simulink model "blimp_state_space"  (R2024b)
settings: Solver=ode113  StartTime=0.0  StopTime=50  RelTol=1e-3
values from neighbouring files (symbols this model uses):
  param = init_params()    [blimp_sim.m]
libraries: slpidlib x1
settings Model: Creator=naikveda
settings SolverCC: SolverResetMethod=Robust

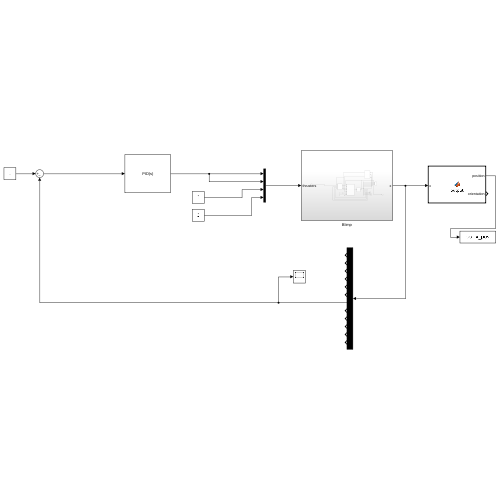
[thumbnail: Simulink's stored preview of the top-level diagram]
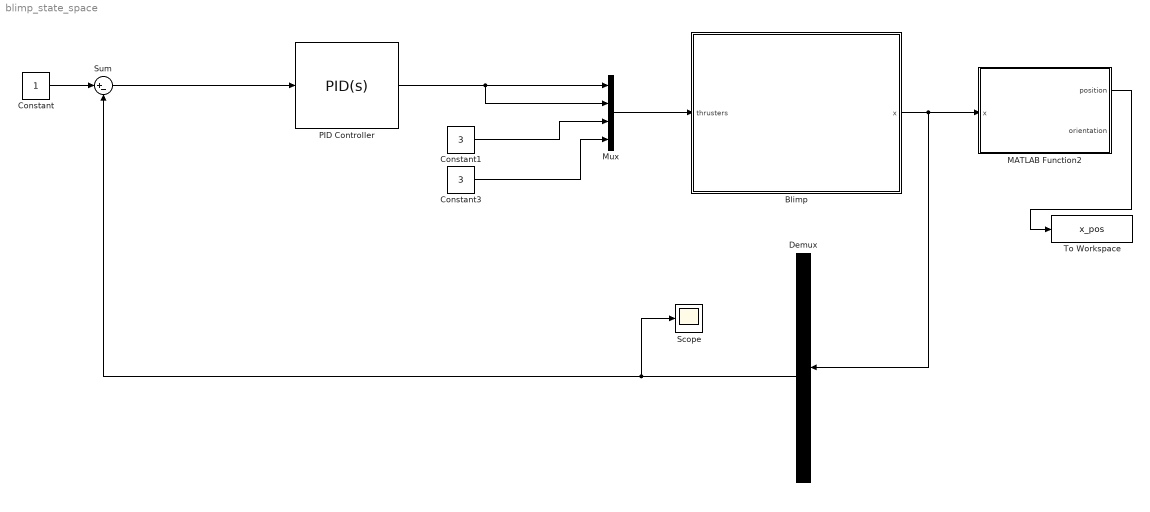
== system blimp_state_space ==
  Blimp : Subsystem
  Constant : Constant
  Constant1 : Constant  Value=3
  Constant3 : Constant  Value=3
  Demux : Demux  Outputs=12
  MATLAB Function2 : MATLAB Function  TreatAsAtomicUnit=on
  Mux : Mux
  PID Controller : slpidlib/PID Controller  Controller=PID  Form=Parallel  TimeDomain=Continuous-time  UseExternalTs=off  SampleTime=-1  IntegratorMethod=Forward Euler  FilterMethod=Forward Euler  ControllerParametersSource=internal  P=1  I=1  UseKiTs=off  D=0  UseExternalDerivativeSource=off  N=100  UseFilter=on  TunerSelectOption=Transfer Function Based (PID Tuner App)  InitialConditionSource=internal  InitialConditionForIntegrator=0  InitialConditionForFilter=0  DifferentiatorICPrevScaledInput=0  ExternalReset=none  TrackingMode=off  Kt=1  LimitOutput=off  SatLimitsSource=internal  UpperSaturationLimit=inf  LowerSaturationLimit=-inf  LinearizeAsGain=on  AntiWindupMode=none  Kb=1  LimitIntegrator=off  UpperIntegratorSaturationLimit=inf  LowerIntegratorSaturationLimit=-inf  POutMin=[]  POutMax=[]  IOutMin=[]  IOutMax=[]  DOutMin=[]  DOutMax=[]  NOutMin=[]  NOutMax=[]  SumOutMin=[]  SumOutMax=[]  SaturationOutMin=[]  SaturationOutMax=[]  PParamMin=[]  PParamMax=[]  IParamMin=[]  IParamMax=[]  DParamMin=[]  DParamMax=[]  NParamMin=[]  NParamMax=[]  KbParamMin=[]  KbParamMax=[]  KtParamMin=[]  KtParamMax=[]  KbOutMin=[]  KbOutMax=[]  KtOutMin=[]  KtOutMax=[]  IntegratorOutMin=[]  IntegratorOutMax=[]  FilterOutMin=[]  FilterOutMax=[]  SumI1OutMin=[]  SumI1OutMax=[]  SumI2OutMin=[]  SumI2OutMax=[]  SumI3OutMin=[]  SumI3OutMax=[]  SumI4OutMin=[]  SumI4OutMax=[]  SumDOutMin=[]  SumDOutMax=[]  DifferentiatorOutMin=[]  DifferentiatorOutMax=[]  FilterDiffOutCoefMin=[]  FilterDiffOutCoefMax=[]  ReciprocalOutMin=[]  ReciprocalOutMax=[]  SumDenOutMin=[]  SumDenOutMax=[]  SumNumOutMin=[]  SumNumOutMax=[]  DivideOutMin=[]  DivideOutMax=[]  UdiffTsProdOutMin=[]  UdiffTsProdOutMax=[]  NTsProdOutMin=[]  NTsProdOutMax=[]  UintegralTsProdOutMin=[]  UintegralTsProdOutMax=[]  UngainTsProdOutMin=[]  UngainTsProdOutMax=[]  ClampingZeroOutDataTypeStr=Inherit: Inherit via back propagation  ClampingZeroOutMin=[]  ClampingZeroOutMax=[]  FilterDenConstantOutDataTypeStr=Inherit: Inherit via back propagation  FilterDenConstantOutMin=[]  FilterDenConstantOutMax=[]  PCopyOutDataTypeStr=Inherit: Inherit via back propagation  PCopyOutMin=[]  PCopyOutMax=[]  NCopyOutDataTypeStr=Inherit: Inherit via back propagation  NCopyOutMin=[]  NCopyOutMax=[]  IntegratorContinuousStateAttributes=''  IntegratorStateMustResolveToSignalObject=off  IntegratorRTWStateStorageClass=Auto  FilterContinuousStateAttributes=''  FilterStateMustResolveToSignalObject=off  FilterRTWStateStorageClass=Auto  ParallelPVariant=InternalParameters  IdealPVariant=Disabled  IVariant=InternalParameters  DVariant=InternalParameters  IntegratorVariant=Continuous  SatVariant=Disabled  AWVariant=Passthrough  PCopyVariant=Disabled  TRVariant=Disabled  FdbkBlocksVariant=Forward  IdealPFdbkVariant=Disabled  SatFdbkVariant=Disabled  DerivativeFilterVariant=ContFilter  NVariant=InternalParameters  NCopyVariant=Disabled  FilterICVariant=InternalICsFilter  IntegratorICVariant=InternalICs  ExternalResetVariant=Disabled  TRSumVariant=Passthrough  SumFdbkVariant=Disabled  SumVariant=Sum_PID  TsampFilterVariant=InternalTs  TsampNgainVariant=Passthrough  TsampIntegralVariant=Disabled_SignalSpec  ExternalSaturationOutDataTypeStr=Inherit: Same as second input  DerivativeSourceVariant=ErrorSignal  PreIntVariant=InternalPreInt
  Scope : Scope
  Sum : Sum  Inputs=|+-
  To Workspace : ToWorkspace  VariableName=x_pos  SaveFormat=Timeseries  SampleTime=-1
  wires:
  MATLAB Function2/1(position) -> To Workspace/1
  Constant1/1 -> Mux/3
  Constant3/1 -> Mux/4
  Mux/1 -> Blimp/1(thrusters)
  Blimp/1(x) -> Demux/1, MATLAB Function2/1(x)
  PID Controller/1 -> Mux/1, Mux/2
  Demux/7 -> Scope/1, Sum/2
  Constant/1 -> Sum/1
  Sum/1 -> PID Controller/1

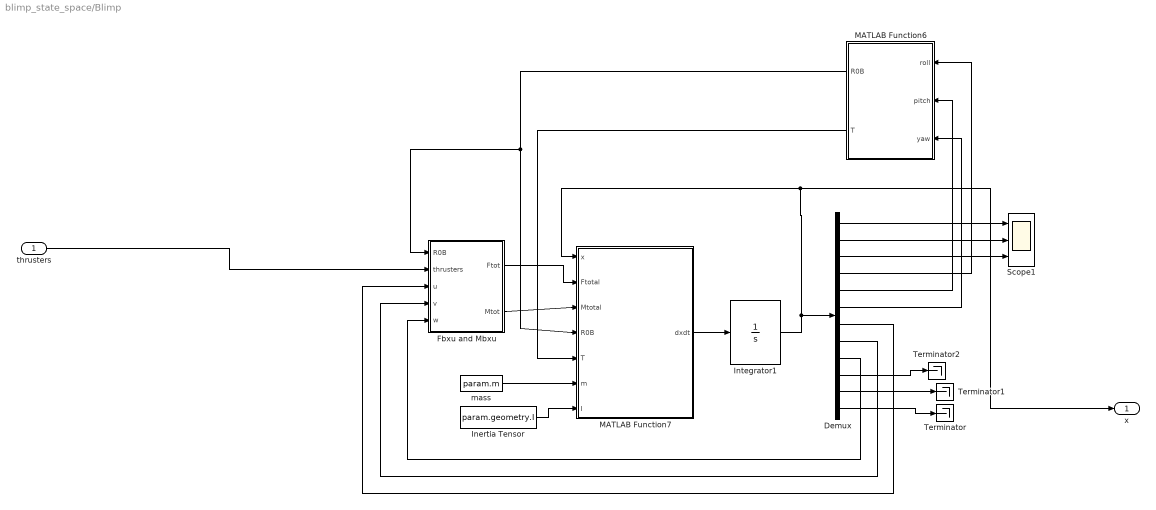
== system blimp_state_space/Blimp ==
  thrusters : Inport
  Demux : Demux  Outputs=12
  Fbxu and Mbxu : Subsystem
  Inertia Tensor : Constant  Value=param.geometry.I  VectorParams1D=off
  Integrator1 : Integrator
  MATLAB Function6 : MATLAB Function  TreatAsAtomicUnit=on
  MATLAB Function7 : MATLAB Function  TreatAsAtomicUnit=on
  Scope1 : Scope  NumInputPorts=3
  Terminator : Terminator
  Terminator1 : Terminator
  Terminator2 : Terminator
  mass : Constant  Value=param.m
  x : Outport
  wires:
  Demux/1 -> Scope1/1
  MATLAB Function6/1(R0B) -> Fbxu and Mbxu/1(R0B), MATLAB Function7/4(R0B)
  MATLAB Function6/2(T) -> MATLAB Function7/5(T)
  Demux/11 -> Terminator1/1
  Demux/5 -> MATLAB Function6/2(pitch)
  Integrator1/1 -> x/1, MATLAB Function7/1(x), Demux/1
  mass/1 -> MATLAB Function7/6(m)
  MATLAB Function7/1(dxdt) -> Integrator1/1
  Demux/9 -> Fbxu and Mbxu/5(w)
  Inertia Tensor/1 -> MATLAB Function7/7(I)
  Demux/10 -> Terminator2/1
  Demux/4 -> MATLAB Function6/1(roll)
  Demux/6 -> MATLAB Function6/3(yaw)
  Demux/12 -> Terminator/1
  Demux/3 -> Scope1/3
  Demux/2 -> Scope1/2
  Fbxu and Mbxu/1(Ftot) -> MATLAB Function7/2(Ftotal)
  Demux/7 -> Fbxu and Mbxu/3(u)
  Demux/8 -> Fbxu and Mbxu/4(v)
  Fbxu and Mbxu/2(Mtot) -> MATLAB Function7/3(Mtotal)
  thrusters/1 -> Fbxu and Mbxu/2(thrusters)

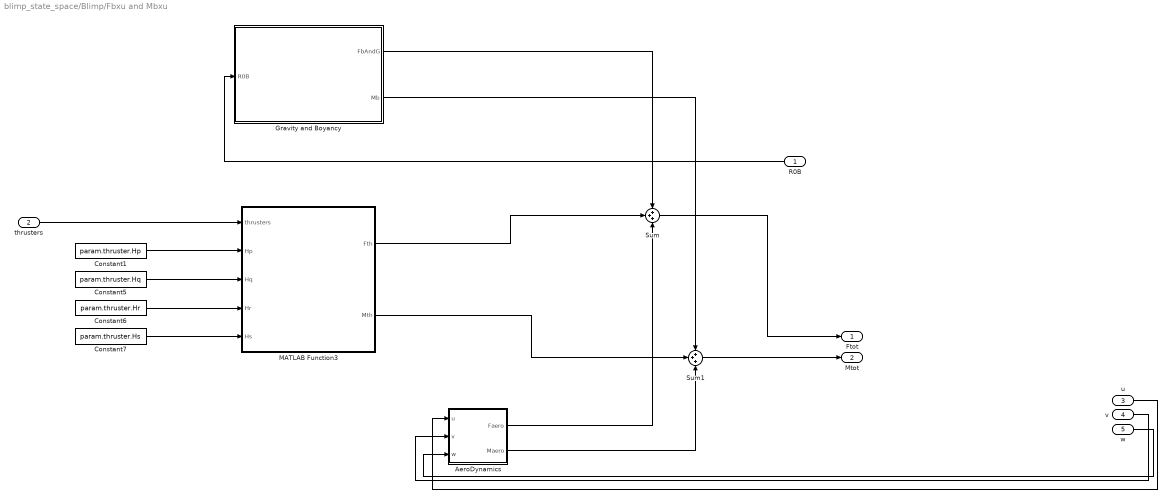
== system blimp_state_space/Blimp/Fbxu and Mbxu ==
  R0B : Inport
  thrusters : Inport  Port=2
  u : Inport  Port=3
  v : Inport  Port=4
  w : Inport  Port=5
  AeroDynamics : Subsystem
  Constant1 : Constant  Value=param.thruster.Hp  VectorParams1D=off
  Constant5 : Constant  Value=param.thruster.Hq  VectorParams1D=off
  Constant6 : Constant  Value=param.thruster.Hr  VectorParams1D=off
  Constant7 : Constant  Value=param.thruster.Hs  VectorParams1D=off
  Gravity and Boyancy : Subsystem
  MATLAB Function3 : MATLAB Function  TreatAsAtomicUnit=on
  Sum : Sum  Inputs=+++
  Sum1 : Sum  Inputs=+++
  Ftot : Outport
  Mtot : Outport  Port=2
  wires:
  Constant1/1 -> MATLAB Function3/2(Hp)
  Constant7/1 -> MATLAB Function3/5(Hs)
  MATLAB Function3/1(Fth) -> Sum/2
  AeroDynamics/2(Maero) -> Sum1/3
  Constant5/1 -> MATLAB Function3/3(Hq)
  MATLAB Function3/2(Mth) -> Sum1/2
  Constant6/1 -> MATLAB Function3/4(Hr)
  AeroDynamics/1(Faero) -> Sum/3
  Gravity and Boyancy/1(FbAndG) -> Sum/1
  Sum/1 -> Ftot/1
  Gravity and Boyancy/2(Mb) -> Sum1/1
  Sum1/1 -> Mtot/1
  thrusters/1 -> MATLAB Function3/1(thrusters)
  w/1 -> AeroDynamics/3(w)
  u/1 -> AeroDynamics/1(u)
  v/1 -> AeroDynamics/2(v)
  R0B/1 -> Gravity and Boyancy/1(R0B)

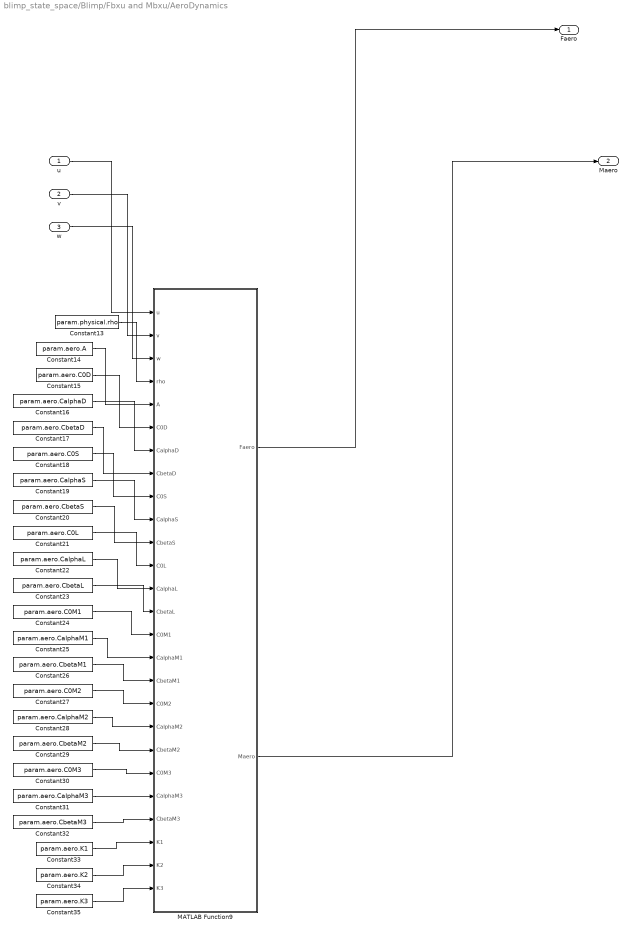
== system blimp_state_space/Blimp/Fbxu and Mbxu/AeroDynamics ==
  u : Inport
  v : Inport  Port=2
  w : Inport  Port=3
  Constant13 : Constant  Value=param.physical.rho
  Constant14 : Constant  Value=param.aero.A
  Constant15 : Constant  Value=param.aero.C0D
  Constant16 : Constant  Value=param.aero.CalphaD
  Constant17 : Constant  Value=param.aero.CbetaD
  Constant18 : Constant  Value=param.aero.C0S
  Constant19 : Constant  Value=param.aero.CalphaS
  Constant20 : Constant  Value=param.aero.CbetaS
  Constant21 : Constant  Value=param.aero.C0L
  Constant22 : Constant  Value=param.aero.CalphaL
  Constant23 : Constant  Value=param.aero.CbetaL
  Constant24 : Constant  Value=param.aero.C0M1
  Constant25 : Constant  Value=param.aero.CalphaM1
  Constant26 : Constant  Value=param.aero.CbetaM1
  Constant27 : Constant  Value=param.aero.C0M2
  Constant28 : Constant  Value=param.aero.CalphaM2
  Constant29 : Constant  Value=param.aero.CbetaM2
  Constant30 : Constant  Value=param.aero.C0M3
  Constant31 : Constant  Value=param.aero.CalphaM3
  Constant32 : Constant  Value=param.aero.CbetaM3
  Constant33 : Constant  Value=param.aero.K1
  Constant34 : Constant  Value=param.aero.K2
  Constant35 : Constant  Value=param.aero.K3
  MATLAB Function9 : MATLAB Function  TreatAsAtomicUnit=on
  Faero : Outport
  Maero : Outport  Port=2
  wires:
  Constant23/1 -> MATLAB Function9/14(CbetaL)
  Constant17/1 -> MATLAB Function9/8(CbetaD)
  Constant18/1 -> MATLAB Function9/9(C0S)
  Constant16/1 -> MATLAB Function9/7(CalphaD)
  Constant13/1 -> MATLAB Function9/4(rho)
  Constant33/1 -> MATLAB Function9/24(K1)
  Constant31/1 -> MATLAB Function9/22(CalphaM3)
  Constant24/1 -> MATLAB Function9/15(C0M1)
  Constant29/1 -> MATLAB Function9/20(CbetaM2)
  MATLAB Function9/2(Maero) -> Maero/1
  Constant22/1 -> MATLAB Function9/13(CalphaL)
  Constant20/1 -> MATLAB Function9/11(CbetaS)
  Constant15/1 -> MATLAB Function9/6(C0D)
  Constant35/1 -> MATLAB Function9/26(K3)
  Constant28/1 -> MATLAB Function9/19(CalphaM2)
  Constant21/1 -> MATLAB Function9/12(C0L)
  Constant32/1 -> MATLAB Function9/23(CbetaM3)
  MATLAB Function9/1(Faero) -> Faero/1
  Constant26/1 -> MATLAB Function9/17(CbetaM1)
  Constant25/1 -> MATLAB Function9/16(CalphaM1)
  Constant30/1 -> MATLAB Function9/21(C0M3)
  Constant14/1 -> MATLAB Function9/5(A)
  Constant19/1 -> MATLAB Function9/10(CalphaS)
  Constant27/1 -> MATLAB Function9/18(C0M2)
  Constant34/1 -> MATLAB Function9/25(K2)
  u/1 -> MATLAB Function9/1(u)
  v/1 -> MATLAB Function9/2(v)
  w/1 -> MATLAB Function9/3(w)

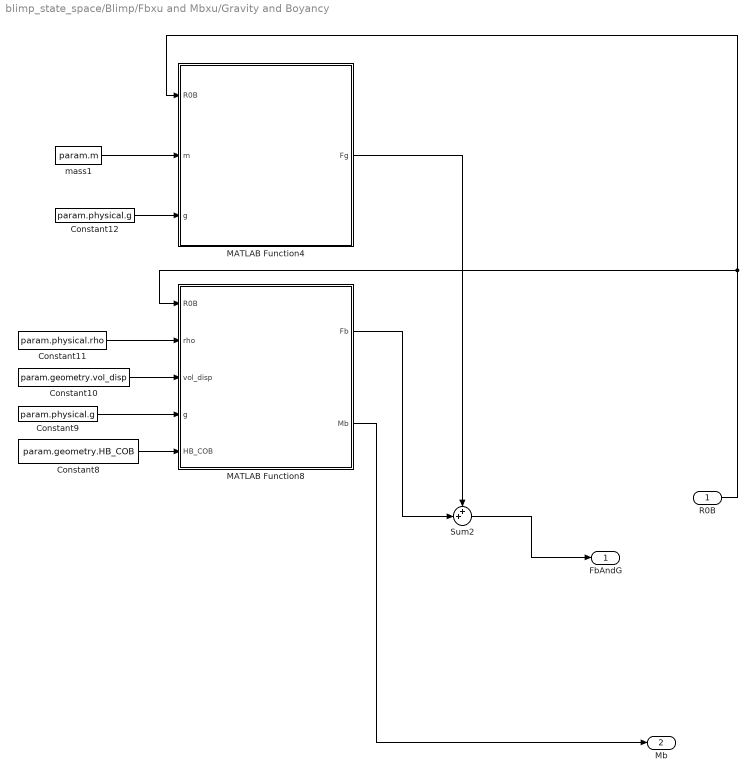
== system blimp_state_space/Blimp/Fbxu and Mbxu/Gravity and Boyancy ==
  R0B : Inport
  Constant10 : Constant  Value=param.geometry.vol_disp
  Constant11 : Constant  Value=param.physical.rho
  Constant12 : Constant  Value=param.physical.g
  Constant8 : Constant  Value=param.geometry.HB_COB  VectorParams1D=off
  Constant9 : Constant  Value=param.physical.g
  MATLAB Function4 : MATLAB Function  TreatAsAtomicUnit=on
  MATLAB Function8 : MATLAB Function  TreatAsAtomicUnit=on
  Sum2 : Sum  Inputs=++|
  mass1 : Constant  Value=param.m
  FbAndG : Outport
  Mb : Outport  Port=2
  wires:
  Constant12/1 -> MATLAB Function4/3(g)
  Constant11/1 -> MATLAB Function8/2(rho)
  MATLAB Function4/1(Fg) -> Sum2/1
  Constant9/1 -> MATLAB Function8/4(g)
  mass1/1 -> MATLAB Function4/2(m)
  Constant8/1 -> MATLAB Function8/5(HB_COB)
  R0B/1 -> MATLAB Function4/1(R0B), MATLAB Function8/1(R0B)
  Constant10/1 -> MATLAB Function8/3(vol_disp)
  MATLAB Function8/1(Fb) -> Sum2/2
  MATLAB Function8/2(Mb) -> Mb/1
  Sum2/1 -> FbAndG/1

== matlab function blimp_state_space/MATLAB Function2 ==
  data: x input; position output; orientation output
function [position, orientation] = output(x)
% OUTPUT Extract position and orientation from state vector
%
% Inputs:
%   x - 12-element state vector with:
%       x(1) = x position
%       x(2) = y position 
%       x(3) = z position
%       x(4) = roll (phi)
%       x(5) = pitch (theta)
%       x(6) = yaw (psi)
%       x(7:12) = velocities and angular rates (not used in this block)
%
% Outputs:
%   position - 3-element vector [x; y; z]
%   orientation - 3-element vector [roll; pitch; yaw] in radians
%
% This function simply extracts the position and orientation components
% from the full state vector for easier visualization and monitoring.

% Extract position (first 3 elements)
position = x(1:3);

% Extract orientation (elements 4-6)
orientation = x(4:6);

% Note: You can add conversions here if needed, for example:
% - Convert radians to degrees
% - Apply coordinate transformations
% - Calculate derived values (e.g., altitude = -z)
end

== matlab function blimp_state_space/Blimp/Fbxu and Mbxu/MATLAB Function3 ==
  data: thrusters input; Fth output; Mth output; Hp input; Hq input; Hr input; Hs input
function [Fth, Mth] = thruster_force(thrusters, Hp, Hq, Hr, Hs)
% THRUSTER_FORCE Calculate thruster forces and moments
%
% Inputs:
%   thrusters - 4-element vector of thruster commands [p; q; r; s]
%   Hp, Hq, Hr, Hs - Thruster position matrices (each 3x4)
%
% Outputs:
%   Fth - Thruster force vector [3x1]
%   Mth - Thruster moment vector [3x1]

% Extract thruster values
u_p = thrusters(1);
u_q = thrusters(2);
u_r = thrusters(3);
u_s = thrusters(4);

% Calculate individual thruster forces
Fth_P = Hp(1:3,1:3)*[0; 0; u_p];
Fth_Q = Hq(1:3,1:3)*[0; 0; u_q];
Fth_R = Hr(1:3,1:3)*[0; 0; u_r];
Fth_S = Hs(1:3,1:3)*[0; 0; u_s];

% Calculate total thrust force
Fth = Fth_P + Fth_Q + Fth_R + Fth_S;

% Calculate thrust moments
Mth = cross(Hp(1:3,4), Fth_P) + ...
      cross(Hq(1:3,4), Fth_Q) + ...
      cross(Hr(1:3,4), Fth_R) + ...
      cross(Hs(1:3,4), Fth_S);
end

== matlab function blimp_state_space/Blimp/Fbxu and Mbxu/Gravity and Boyancy/MATLAB Function4 ==
  data: R0B input; Fg output; m input; g input
function Fg = gravity_force(R0B, m, g)

Fg = R0B * [0; 0; -m*g];
end

== matlab function blimp_state_space/Blimp/MATLAB Function6 ==
  data: roll input; R0B output; T output; pitch input; yaw input
function [R0B, T] = kinematics_transform(roll, pitch, yaw)

% Calculate transformation matrix for angular velocities
T = [cos(yaw)*cos(pitch), -sin(yaw), 0;
     sin(yaw)*cos(pitch), cos(yaw), 0;
     -sin(pitch), 0, 1];

% Calculate rotation matrix from inertial to body frame
R0B = [cos(pitch)*cos(yaw), cos(yaw)*sin(roll)*sin(pitch)-cos(roll)*sin(yaw), cos(roll)*cos(yaw)*sin(pitch)+sin(roll)*sin(yaw);
       cos(pitch)*sin(yaw), cos(roll)*cos(yaw)-sin(roll)*sin(pitch)*sin(yaw), cos(roll)*sin(pitch)*sin(yaw)-sin(roll)*sin(yaw);
       -sin(pitch), cos(pitch)*sin(roll), cos(roll)*cos(pitch)];
end

== matlab function blimp_state_space/Blimp/MATLAB Function7 ==
  data: x input; dxdt output; Ftotal input; Mtotal input; R0B input; T input; m input; I input
function dxdt = state_derivatives(x, Ftotal, Mtotal, R0B, T, m, I)
% STATE_DERIVATIVES Calculate state derivatives from forces and moments
%
% Inputs:
%   x - State vector [12x1]
%   Ftotal - Total force vector in body frame [3x1]
%   Mtotal - Total moment vector in body frame [3x1]
%   R0B - Rotation matrix from inertial to body frame [3x3]
%   T - Angular velocity transformation matrix [3x3]
%   m - Mass [scalar]
%   I - Inertia matrix [3x3]
%
% Outputs:
%   dxdt - State derivative vector [12x1]

% Initialize state derivative vector
dxdt = zeros(12, 1);

% Position derivatives (x, y, z)
dxdt(1:3) = R0B*x(7:9);

% Attitude derivatives (roll, pitch, yaw)
dxdt(4:6) = (T^(-1))*R0B*x(10:12);

% Linear velocity derivatives (u, v, w)
dxdt(7:9) = (1/m)*(Ftotal - m*(cross(x(10:12),x(7:9))));

% Angular velocity derivatives (p, q, r)
dxdt(10:12) = (I^(-1))*(Mtotal - cross(x(10:12),(I*x(10:12))));
end

== matlab function blimp_state_space/Blimp/Fbxu and Mbxu/Gravity and Boyancy/MATLAB Function8 ==
  data: R0B input; Fb output; rho input; vol_disp input; g input; HB_COB input; Mb output
function [Fb, Mb] = buoyancy_force(R0B, rho, vol_disp, g, HB_COB)

% Calculate buoyancy force in body frame
Fb = R0B * [0; 0; rho*vol_disp*g];

% Calculate buoyancy moment
Mb = cross(HB_COB(1:3,4), Fb);
end

== matlab function blimp_state_space/Blimp/Fbxu and Mbxu/AeroDynamics/MATLAB Function9 ==
  data: u input; v input; w input; Faero output; rho input; A input; Maero output; C0D input; CalphaD input; CbetaD input; C0S input; CalphaS input; CbetaS input; C0L input; CalphaL input; CbetaL input; C0M1 input; CalphaM1 input; CbetaM1 input; C0M2 input; CalphaM2 input; CbetaM2 input; C0M3 input; CalphaM3 input; CbetaM3 input; K1 input; K2 input; K3 input
function [Faero, Maero] = aero_force_vector(u, v, w, rho, A, C0D, CalphaD, CbetaD, C0S, CalphaS, CbetaS, C0L, CalphaL, CbetaL, C0M1, CalphaM1, CbetaM1, C0M2, CalphaM2, CbetaM2, C0M3, CalphaM3, CbetaM3, K1, K2, K3)
    
    Rbb = [1 0 0; 0 -1 0; 0 0 -1];
    velA = Rbb*[u;v;w];    
    V = norm(velA);

    if velA <= 0.01
        Faero = zeros(3,1);
        Maero = zeros(3,1);
    else

        ua = velA(1);
        va = velA(2);
        wa = velA(3);

        attack_angle = atan(wa/ua);
        sideslip_angle = asin(va/V);
    
    RBV = [[cos(attack_angle)*cos(sideslip_angle), -cos(attack_angle)*sin(sideslip_angle),  -sin(attack_angle)]
                          [sin(sideslip_angle),  cos(sideslip_angle), 0]
                          [sin(attack_angle)*cos(sideslip_angle), -sin(attack_angle)*sin(sideslip_angle), cos(attack_angle)]];
    
    Cd = C0D + CalphaD*attack_angle^2 + CbetaD*sideslip_angle^2;
    Cs = C0S + CalphaS*attack_angle^2 + CbetaS*sideslip_angle;
    Cl = C0L + CalphaL*attack_angle + CbetaL*sideslip_angle^2;

    Cm1 = C0M1 + CalphaM1*attack_angle + CbetaM1*sideslip_angle;
    Cm2 = C0M2 + CalphaM2*attack_angle + CbetaM2*sideslip_angle^4;
    Cm3 = C0M3 + CalphaM3*attack_angle + CbetaM3*sideslip_angle;
    
    
    D = (0.5)*rho*V*V*A*Cd;
    S = (0.5)*rho*V*V*A*Cs;
    L = (0.5)*rho*V*V*A*Cl;

    M1 = (0.5)*rho*V*V*A*Cm1 + K1*0;
    M2 = (0.5)*rho*V*V*A*Cm2 + K2*0;
    M3 = (0.5)*rho*V*V*A*Cm3 + K3*0;
    Faero = Rbb*RBV * [-D; S; -L];

    Maero = Rbb*RBV * [M1; M2; M3];
    end
